simulink model "FullBridge_BipolarModulation"  (R2021b)
settings: Solver=FixedStepDiscrete  StartTime=0.0  StopTime=0.3  RelTol=1e-3
libraries: spsMosfetLib x4, spsSeriesRLCBranchLib x3, spsVoltageMeasurementLib x2, spsCurrentMeasurementLib x1, spsDCVoltageSourceLib x1, spsTriangleGeneratorLib x1, spspowerguiLib x1
settings Model: Creator=ycay  LastModifiedBy=ycay
settings DataIOCC: ReturnWorkspaceOutputs=off

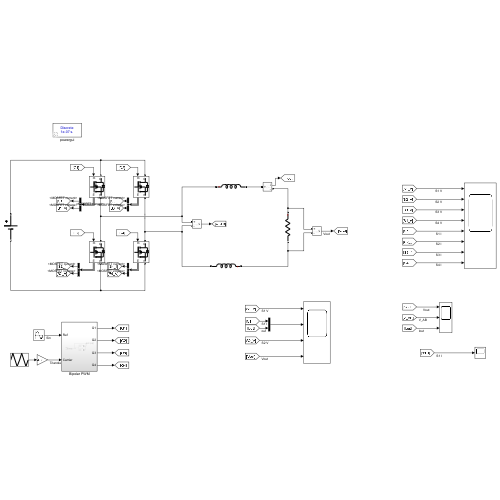
[thumbnail: Simulink's stored preview of the top-level diagram]
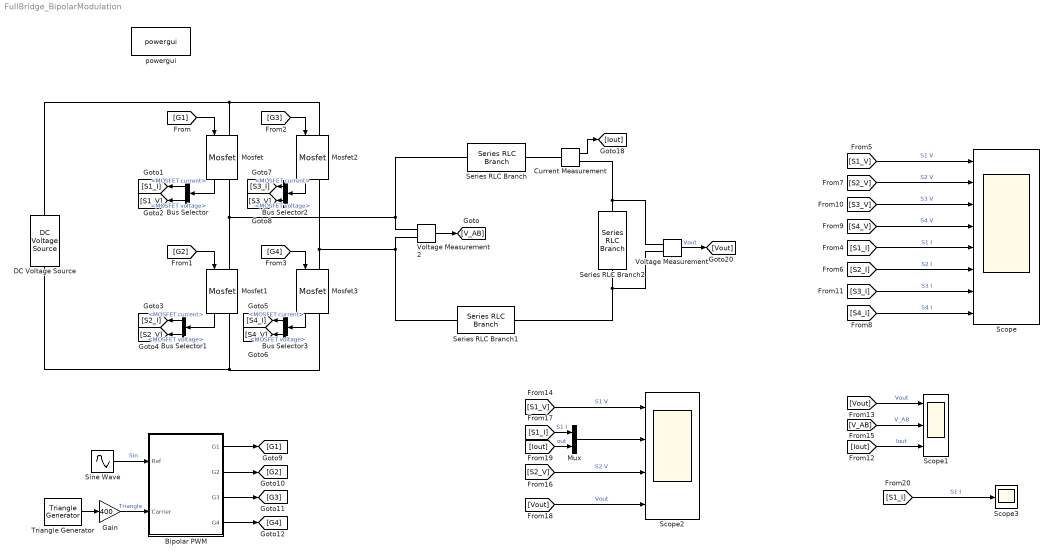
== system FullBridge_BipolarModulation ==
  Bipolar PWM : Subsystem
  Bus Selector{,1..3} (4 alike) : BusSelector  OutputSignals=MOSFET current,MOSFET voltage
  Current Measurement : spsCurrentMeasurementLib/Current Measurement  PhasorSimulation=off  OutputType=Complex  PSBequivalent=0
  DC Voltage Source : spsDCVoltageSourceLib/DC Voltage Source  Amplitude=400  Measurements=None
  Gain : Gain  Gain=400
  Mosfet{,1..3} (4 alike) : spsMosfetLib/Mosfet  Ron=0.001  Lon=0  Rd=0.001  Vfd=0  IC=0  Rs=1e5  Cs=inf  Measurements=on
  Mux : Mux  Inputs=2
  Scope : Scope  NumInputPorts=8
  Scope1 : Scope  NumInputPorts=3
  Scope2 : Scope  NumInputPorts=4
  Scope3 : Scope
  Series RLC Branch : spsSeriesRLCBranchLib/Series RLC Branch  LConnTagsString=__new0  RConnTagsString=__new0  BranchType=L  Resistance=1  Inductance=10e-3  SetiL0=off  InitialCurrent=0  Capacitance=1e-6  Setx0=off  InitialVoltage=0  Measurements=None
  Series RLC Branch1 : spsSeriesRLCBranchLib/Series RLC Branch  LConnTagsString=__new0  RConnTagsString=__new0  BranchType=L  Resistance=1  Inductance=10e-3  SetiL0=off  InitialCurrent=0  Capacitance=1e-6  Setx0=off  InitialVoltage=0  Measurements=None
  Series RLC Branch2 : spsSeriesRLCBranchLib/Series RLC Branch  LConnTagsString=__new0  RConnTagsString=__new0  BranchType=R  Resistance=9  Inductance=1e-3  SetiL0=off  InitialCurrent=0  Capacitance=1e-6  Setx0=off  InitialVoltage=0  Measurements=None
  Sine Wave : Sin  Amplitude=230*sqrt(2)  Frequency=2*pi*50  SampleTime=1e-6
  Triangle Generator : spsTriangleGeneratorLib/Triangle Generator  Freq=1e5  Phase=90  Ts=1e-7
  Voltage Measurement : spsVoltageMeasurementLib/Voltage Measurement  PhasorSimulation=off  OutputType=Complex  PSBequivalent=0
  Voltage Measurement2 : spsVoltageMeasurementLib/Voltage Measurement  PhasorSimulation=off  OutputType=Complex  PSBequivalent=0
  powergui : spspowerguiLib/powergui  Priority=1  SimulationMode=Discrete  SampleTime=1e-7  frequency=60  Iterations=50  frequencyindice=0  Pbase=100e6  ErrMax=1e-4  UnitsV=kV  UnitsW=MW  buscounter=0  FunctionMessages=off  echomessages=off  EnableUseOfTLC=off  CurrentSourceSwitches=off  DisableSnubberDevices=off  DisableRonSwitches=off  DisableVfSwitches=off  DisplayEquations=off  AutomaticDiscreteSolvers=off  SolverType=Tustin/Backward Euler (TBE)  Interpol=off  ExternalGateDelay=off  methode=off  Ts=100  x0status=blocks  SPID=on  SwTol=0  HookPort=off  NonlinearTolerance=1e-4  nMaxIteration=100  ContinueOnMaxIteration=off  RestoreLinks=warning  ResistiveCurrentMeasurement=off  Frange=[0:2:500]  Ylog=off  Xlog=on  ShowGrid=off  save=off  variable=ZData  structure=0  ZoomFFT=off  StartTime=0.0  cycles=1  DisplayStyle=1  fundamental=60  FreqAxis=off  MaxFrequency=1000  frequencyindicesteady=1  RmsSteady=1  display=off
  wires:
  Voltage Measurement/1 -> [Vout]  "Vout"
  [G1] -> Mosfet/1
  Current Measurement/1 -> [Iout]
  Voltage Measurement2/1 -> [V_AB]
  [G3] -> Mosfet2/1
  [G4] -> Mosfet3/1
  [G2] -> Mosfet1/1
  Mosfet/1 -> Bus Selector/1
  Mosfet1/1 -> Bus Selector1/1
  Mosfet2/1 -> Bus Selector2/1
  Mosfet3/1 -> Bus Selector3/1
  Bus Selector/1 -> [S1_I]  "<MOSFET current>"
  Bus Selector/2 -> [S1_V]  "<MOSFET voltage>"
  Bus Selector1/2 -> [S2_V]  "<MOSFET voltage>"
  Bus Selector1/1 -> [S2_I]  "<MOSFET current>"
  Bus Selector3/2 -> [S4_V]  "<MOSFET voltage>"
  Bus Selector3/1 -> [S4_I]  "<MOSFET current>"
  Bus Selector2/2 -> [S3_V]  "<MOSFET voltage>"
  Bus Selector2/1 -> [S3_I]  "<MOSFET current>"
  [S1_V] -> Scope/1  "S1 V"
  [S2_V] -> Scope/2  "S2 V"
  [S3_V] -> Scope/3  "S3 V"
  [S4_V] -> Scope/4  "S4 V"
  [S1_I] -> Scope/5  "S1 I"
  [S2_I] -> Scope/6  "S2 I"
  [S3_I] -> Scope/7  "S3 I"
  [S4_I] -> Scope/8  "S4 I"
  Bipolar PWM/2(G2) -> [G2]
  Gain/1 -> Bipolar PWM/2(Carrier)  "Triangle"
  Bipolar PWM/1(G1) -> [G1]
  Bipolar PWM/3(G3) -> [G3]
  Sine Wave/1 -> Bipolar PWM/1(Ref)  "Sin"
  Bipolar PWM/4(G4) -> [G4]
  Triangle Generator/1 -> Gain/1
  [Vout] -> Scope1/1  "Vout"
  [V_AB] -> Scope1/2  "V_AB"
  [Iout] -> Scope1/3  "Iout"
  [S1_V] -> Scope2/1  "S1 V"
  [S2_V] -> Scope2/3  "S2 V"
  [Vout] -> Scope2/4  "Vout"
  Mux/1 -> Scope2/2
  [S1_I] -> Mux/1  "S1 I"
  [Iout] -> Mux/2  "out"
  [S1_I] -> Scope3/1  "S1 I"
  connections:
  DC Voltage Source/LConn1 -- Mosfet1/RConn1 -- Mosfet3/RConn1
  Voltage Measurement/LConn2 -- Series RLC Branch1/LConn1 -- Series RLC Branch2/RConn1
  Mosfet1/LConn1 -- Mosfet/RConn1 -- Voltage Measurement2/LConn1 -- Series RLC Branch/LConn1
  Series RLC Branch2/LConn1 -- Current Measurement/RConn1 -- Voltage Measurement/LConn1
  Mosfet2/LConn1 -- Mosfet/LConn1 -- DC Voltage Source/RConn1
  Series RLC Branch/RConn1 -- Current Measurement/LConn1
  Series RLC Branch1/RConn1 -- Mosfet3/LConn1 -- Mosfet2/RConn1 -- Voltage Measurement2/LConn2

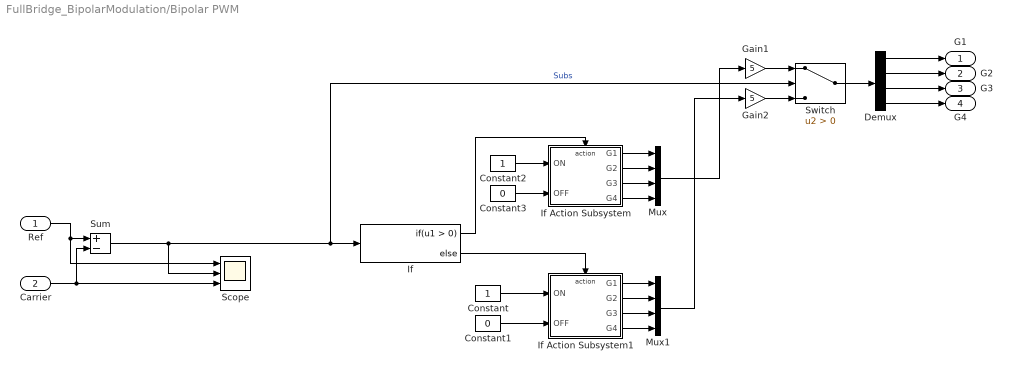
== system FullBridge_BipolarModulation/Bipolar PWM ==
  Ref : Inport
  Carrier : Inport  Port=2
  Constant : Constant
  Constant1 : Constant  Value=0
  Constant2 : Constant
  Constant3 : Constant  Value=0
  Demux : Demux
  Gain1 : Gain  Gain=5
  Gain2 : Gain  Gain=5
  If : If
  If Action Subsystem : Subsystem  TreatAsAtomicUnit=on
  If Action Subsystem1 : Subsystem  TreatAsAtomicUnit=on
  Mux : Mux
  Mux1 : Mux
  Scope : Scope  NumInputPorts=3
  Sum : Sum  Inputs=+-
  Switch : Switch  Criteria=u2 > Threshold
  G1 : Outport
  G2 : Outport  Port=2
  G3 : Outport  Port=3
  G4 : Outport  Port=4
  wires:
  If/2 -> If Action Subsystem1/Action
  If Action Subsystem/2(G2) -> Mux/2
  Constant/1 -> If Action Subsystem1/1(ON)
  Switch/1 -> Demux/1
  Mux/1 -> Gain1/1
  Constant3/1 -> If Action Subsystem/2(OFF)
  If/1 -> If Action Subsystem/Action
  Sum/1 -> Switch/2, If/1, Scope/2  "Subs"
  If Action Subsystem/1(G1) -> Mux/1
  If Action Subsystem1/4(G4) -> Mux1/4
  Constant2/1 -> If Action Subsystem/1(ON)
  If Action Subsystem/4(G4) -> Mux/4
  If Action Subsystem1/3(G3) -> Mux1/3
  Gain2/1 -> Switch/3
  If Action Subsystem/3(G3) -> Mux/3
  If Action Subsystem1/1(G1) -> Mux1/1
  Mux1/1 -> Gain2/1
  If Action Subsystem1/2(G2) -> Mux1/2
  Gain1/1 -> Switch/1
  Constant1/1 -> If Action Subsystem1/2(OFF)
  Demux/4 -> G4/1
  Demux/3 -> G3/1
  Demux/2 -> G2/1
  Demux/1 -> G1/1
  Ref/1 -> Scope/1, Sum/1
  Carrier/1 -> Sum/2, Scope/3

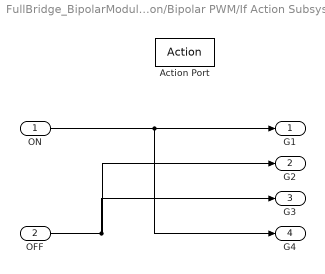
== system FullBridge_BipolarModulation/Bipolar PWM/If Action Subsystem ==
  ON : Inport
  OFF : Inport  Port=2
  Action Port : ActionPort  ActionPortLabel=if(u1 > 0)
  G1 : Outport
  G2 : Outport  Port=2
  G3 : Outport  Port=3
  G4 : Outport  Port=4
  wires:
  ON/1 -> G4/1, G1/1
  OFF/1 -> G3/1, G2/1

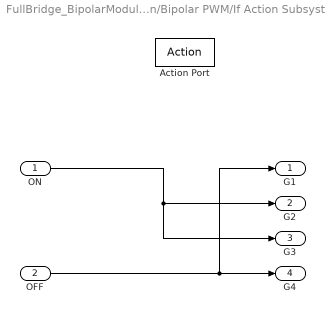
== system FullBridge_BipolarModulation/Bipolar PWM/If Action Subsystem1 ==
  ON : Inport
  OFF : Inport  Port=2
  Action Port : ActionPort  ActionPortLabel=else
  G1 : Outport
  G2 : Outport  Port=2
  G3 : Outport  Port=3
  G4 : Outport  Port=4
  wires:
  ON/1 -> G2/1, G3/1
  OFF/1 -> G4/1, G1/1
